simulink model "conmutador22"  (Simulink 7.1)
settings: Solver=ode45  StartTime=0.0  StopTime=10.0  RelTol=1e-3
libraries: simeventsrouting1 x8, simeventssink1 x4, simeventsqueue1 x2, simeventsattributes2 x2, simeventsgates1 x2
settings Model: Creator=EmP  LastModifiedBy=EmP
settings SimEventsCC: propLogEventsScheduled=0  propLogEventsExecuted=0  propLogDepartureEvents=0  propDisplayEventCalendar=0  propDiagAttribOutput=1  propDiagFcnCallOutput=1  propDiagStatOutput=0

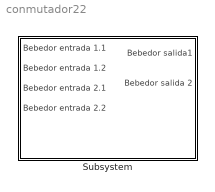
== system conmutador22 ==
  Subsystem : Subsystem

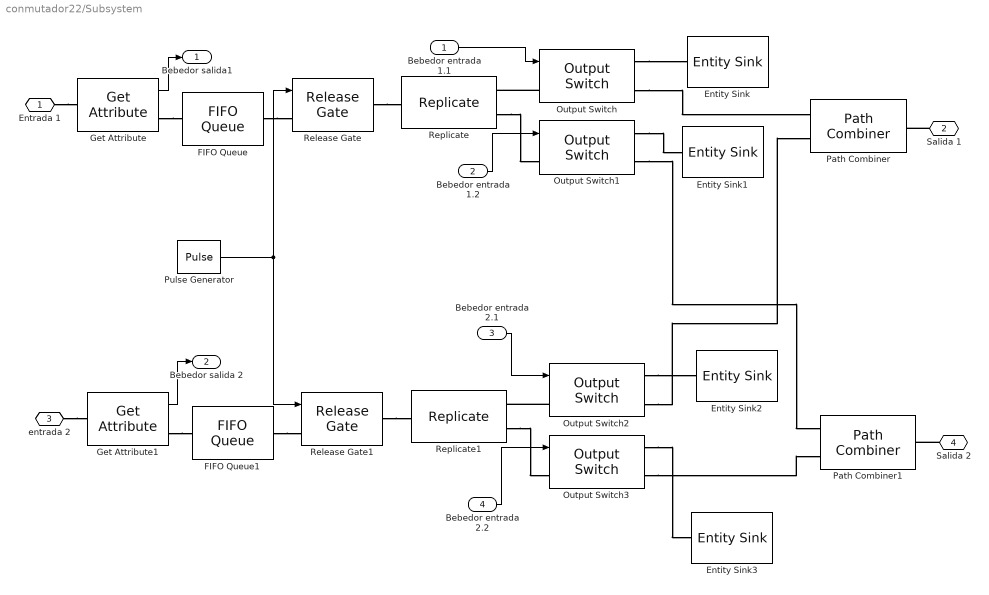
== system conmutador22/Subsystem ==
  Bebedor entrada 1.1 : Inport
  Bebedor entrada 1.2 : Inport  Port=2
  Bebedor entrada 2.1 : Inport  Port=3
  Bebedor entrada 2.2 : Inport  Port=4
  Entity Sink{,1..3} (4 alike) : simeventssink1/Entity Sink  Priority=1  SystemSampleTime=-1  AvailableForArrivals=on  StatNumberArrived=Off
  FIFO Queue : simeventsqueue1/FIFO Queue  Priority=1  SystemSampleTime=-1  Capacity=25  EnableTOPort=off  StatNumberDeparted=Off  StatNumberInBlock=Off  StatPendingEntity=Off  StatAverageWait=Off  StatAverageQueueLength=Off  StatNumberTimedout=Off
  FIFO Queue1 : simeventsqueue1/FIFO Queue  Priority=1  SystemSampleTime=-1  Capacity=25  EnableTOPort=off  StatNumberDeparted=Off  StatNumberInBlock=Off  StatPendingEntity=Off  StatAverageWait=Off  StatAverageQueueLength=Off  StatNumberTimedout=Off
  Get Attribute : simeventsattributes2/Get Attribute  Priority=1  DialogController=des_ddg_create  DialogControllerArgs=DataTag7  SystemSampleTime=-1  AttributeName=Attribute1  AttributeMissing=Error  AttributeDefaultValue=1  AttributeSendTiming=After entity departure  AttributeTreatAsVector=1  StatNumberDeparted=Off  EvaluatedDefaultAttributeValue={[]}
  Get Attribute1 : simeventsattributes2/Get Attribute  Priority=1  DialogController=des_ddg_create  DialogControllerArgs=DataTag9  SystemSampleTime=-1  AttributeName=Attribute1  AttributeMissing=Error  AttributeDefaultValue=1  AttributeSendTiming=After entity departure  AttributeTreatAsVector=1  StatNumberDeparted=Off  EvaluatedDefaultAttributeValue={[]}
  Output Switch{,1..3} (4 alike) : simeventsrouting1/Output Switch  Priority=1  SystemSampleTime=-1  NumberOutputPorts=2  SwitchingCriterion=From signal port p  InitialSeed=34567  AttributeName=Attribute1  InitialConditionsOpt=off  InitialConditions=1  EntityBufferOpt=off  SpecifyEventPriority=off  PriorityOutputSwitchSelectPort=4100  TimeoutPortOpt=off  StatNumberDeparted=Off  StatNumberTimedOut=Off  StatPendingEntity=Off  StatLastDeparturePort=Off  EvaluatedNumPorts=2
  Path Combiner : simeventsrouting1/Path Combiner  Priority=1  SystemSampleTime=-1  NumberInputPorts=2  InputPortPrecedence=IN1 port  InitialSeed=45675  SpecifyEventPriority=off  PriorityPathCombinerPortPrecedenceSelection=4100  StatNumberDeparted=Off  StatLastArrivalPort=Off  EvaluatedNumPorts=2
  Path Combiner1 : simeventsrouting1/Path Combiner  Priority=1  SystemSampleTime=-1  NumberInputPorts=2  InputPortPrecedence=IN1 port  InitialSeed=45675  SpecifyEventPriority=off  PriorityPathCombinerPortPrecedenceSelection=4100  StatNumberDeparted=Off  StatLastArrivalPort=Off  EvaluatedNumPorts=2
  Pulse Generator : DiscretePulseGenerator  PulseType=Time based  PulseWidth=50
  Release Gate : simeventsgates1/Release Gate  Priority=1  SystemSampleTime=-1  OpenGateUpon=Change in signal from port vc  SignalEdgeOption=Rising  SpecifyEventPriority=off  PriorityGateRelease=2200  StatNumberDeparted=Off
  Release Gate1 : simeventsgates1/Release Gate  Priority=1  SystemSampleTime=-1  OpenGateUpon=Change in signal from port vc  SignalEdgeOption=Rising  SpecifyEventPriority=off  PriorityGateRelease=2200  StatNumberDeparted=Off
  Replicate : simeventsrouting1/Replicate  Priority=1  SystemSampleTime=-1  NumberOutputPorts=2  ReplicateEntityWhen=All entity output ports are not blocked  OutputPortPrecedence=OUT1 port  InitialSeed=56789  ActionUponBlocking=Discard entity  StatNumberArrived=Off  StatNumberDeparted=Off  EvaluatedNumPorts=2
  Replicate1 : simeventsrouting1/Replicate  Priority=1  SystemSampleTime=-1  NumberOutputPorts=2  ReplicateEntityWhen=All entity output ports are not blocked  OutputPortPrecedence=OUT1 port  InitialSeed=56789  ActionUponBlocking=Discard entity  StatNumberArrived=Off  StatNumberDeparted=Off  EvaluatedNumPorts=2
  Entrada 1 : PMIOPort  Port=1  Side=Left
  Salida 1 : PMIOPort  Orientation=left  Port=2  Side=Right
  entrada 2 : PMIOPort  Port=3  Side=Left
  Salida 2 : PMIOPort  Orientation=left  Port=4  Side=Right
  Bebedor salida1 : Outport
  Bebedor salida 2 : Outport  Port=2
  wires:
  Bebedor entrada 1.1/1 -> Output Switch/1
  Get Attribute/1 -> Bebedor salida1/1
  Pulse Generator/1 -> Release Gate/1, Release Gate1/1
  Bebedor entrada 1.2/1 -> Output Switch1/1
  Bebedor entrada 2.1/1 -> Output Switch2/1
  Get Attribute1/1 -> Bebedor salida 2/1
  Bebedor entrada 2.2/1 -> Output Switch3/1
  connections:
  Output Switch/RConn1 -- Entity Sink/LConn1
  Output Switch1/RConn1 -- Entity Sink1/LConn1
  Output Switch2/RConn1 -- Entity Sink2/LConn1
  Output Switch3/RConn1 -- Entity Sink3/LConn1
  Get Attribute/RConn1 -- FIFO Queue/LConn1
  FIFO Queue/RConn1 -- Release Gate/LConn1
  Get Attribute1/RConn1 -- FIFO Queue1/LConn1
  FIFO Queue1/RConn1 -- Release Gate1/LConn1
  Output Switch/LConn1 -- Replicate/RConn1
  Output Switch/RConn2 -- Path Combiner/LConn1
  Replicate/RConn2 -- Output Switch1/LConn1
  Output Switch1/RConn2 -- Path Combiner1/LConn1
  Output Switch2/LConn1 -- Replicate1/RConn1
  Output Switch2/RConn2 -- Path Combiner/LConn2
  Replicate1/RConn2 -- Output Switch3/LConn1
  Output Switch3/RConn2 -- Path Combiner1/LConn2
  Release Gate/RConn1 -- Replicate/LConn1
  Release Gate1/RConn1 -- Replicate1/LConn1
  Entrada 1/RConn1 -- Get Attribute/LConn1
  Salida 1/RConn1 -- Path Combiner/RConn1
  entrada 2/RConn1 -- Get Attribute1/LConn1
  Salida 2/RConn1 -- Path Combiner1/RConn1
